simulink model "ASK"  (R2016a)
settings: Solver=FixedStepDiscrete  StartTime=0.0  StopTime=0.25  FixedStep=1/2000000  RelTol=1e-3
libraries: dsparch4 x4
settings Model: Creator=camj3302  LastModifiedBy=camj3302
settings SolverCC: AutoInsertRateTranBlk=on

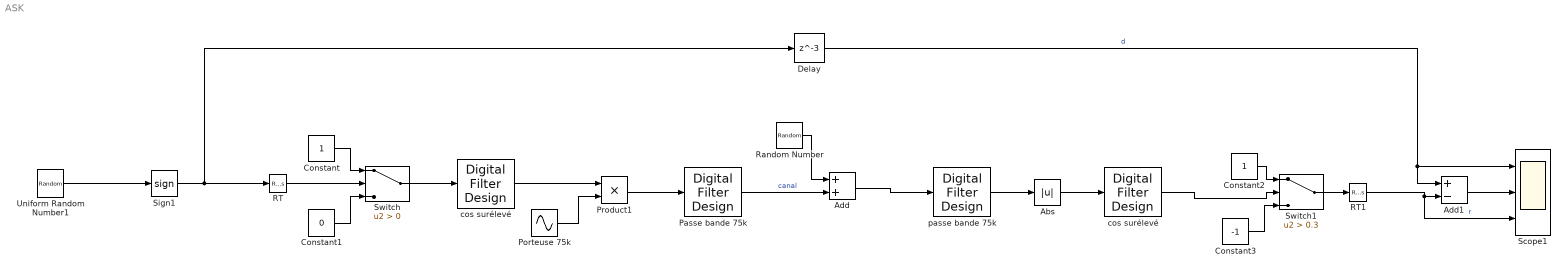
== system ASK ==
  Abs : Abs
  Add : Sum
  Add1 : Sum  Inputs=+-
  Constant : Constant  SampleTime=-1
  Constant1 : Constant  Value=0  SampleTime=-1
  Constant2 : Constant  SampleTime=-1
  Constant3 : Constant  Value=-1  SampleTime=-1
  Delay : Delay  DelayLength=3  InitialCondition=0
  Passe bande 75k : dsparch4/Digital Filter Design  mwdsp_browser_bugfix_var=off
  Porteuse 75k : Sin  Frequency=75000*2*pi  SampleTime=1/2000000
  Product1 : Product
  RT : RateTransition  OutPortSampleTime=5e-07
  RT1 : RateTransition  OutPortSampleTime=1/1000
  Random Number : RandomNumber  Variance=2  SampleTime=1/2000000
  Scope1 : Scope  NumInputPorts=3
  Sign1 : Signum
  Switch : Switch  Criteria=u2 > Threshold
  Switch1 : Switch  Criteria=u2 > Threshold  Threshold=0.3
  Uniform Random Number1 : UniformRandomNumber  SampleTime=1/1000
  cos surélevé : dsparch4/Digital Filter Design  mwdsp_browser_bugfix_var=off
  "cos surélevé " : dsparch4/Digital Filter Design  mwdsp_browser_bugfix_var=off
  passe bande 75k : dsparch4/Digital Filter Design  mwdsp_browser_bugfix_var=off
  wires:
  Product1/1 -> Passe bande 75k/1
  Abs/1 -> "cos surélevé "/1
  Delay/1 -> Scope1/1, Add1/1  "d"
  Switch1/1 -> RT1/1
  Switch/1 -> cos surélevé/1
  Constant1/1 -> Switch/3
  Constant/1 -> Switch/1
  Sign1/1 -> Delay/1, RT/1
  cos surélevé/1 -> Product1/1
  Porteuse 75k/1 -> Product1/2
  passe bande 75k/1 -> Abs/1
  Constant3/1 -> Switch1/3
  Constant2/1 -> Switch1/1
  "cos surélevé "/1 -> Switch1/2
  Passe bande 75k/1 -> Add/2  "canal"
  Uniform Random Number1/1 -> Sign1/1
  RT/1 -> Switch/2
  RT1/1 -> Scope1/3, Add1/2  "r"
  Add1/1 -> Scope1/2
  Random Number/1 -> Add/1
  Add/1 -> passe bande 75k/1
